simulink model "ver2_real_disc"  (R2018b)
settings: Solver=FixedStepAuto  StartTime=0.0  StopTime=10  FixedStep=10e-5  RelTol=1e-3
InitFcn:
  | ver2_real_pend_disc
values from neighbouring files (symbols this model uses):
  A_new = [A,zeros(2,1) ... (first row only)    [ver1_real_pend_cont.m]    (also in ver1_real_pendulum.m; ver2_real_pend_disc.m)
  B_new = [B ... (first row only)    [ver1_real_pend_cont.m]    (also in ver1_real_pendulum.m; ver2_real_pend_disc.m)
  E = [0 ... (first row only)    [ver1_real_pend_cont.m]    (also in ver1_real_pendulum.m; ver2_real_pend_disc.m)
  Init_condition = [0 ... (first row only)    [ver1_real_pend_cont.m]    (also in ver1_real_pendulum.m; ver2_real_pend_disc.m)
  K = lqr(A_new,B_new,Q,R)    [ver1_real_pend_cont.m]    (also in ver1_real_pendulum.m = dlqr(A_new,B_new,Q,R); ver2_real_pend_disc.m = dlqr(A_ne,B_ne,Q,R))
settings Model: Creator=Mehmet  LastModifiedBy=Seko
settings SFSimCC: SimUseLocalCustomCode=off
settings RTWCC: RTWUseLocalCustomCode=off

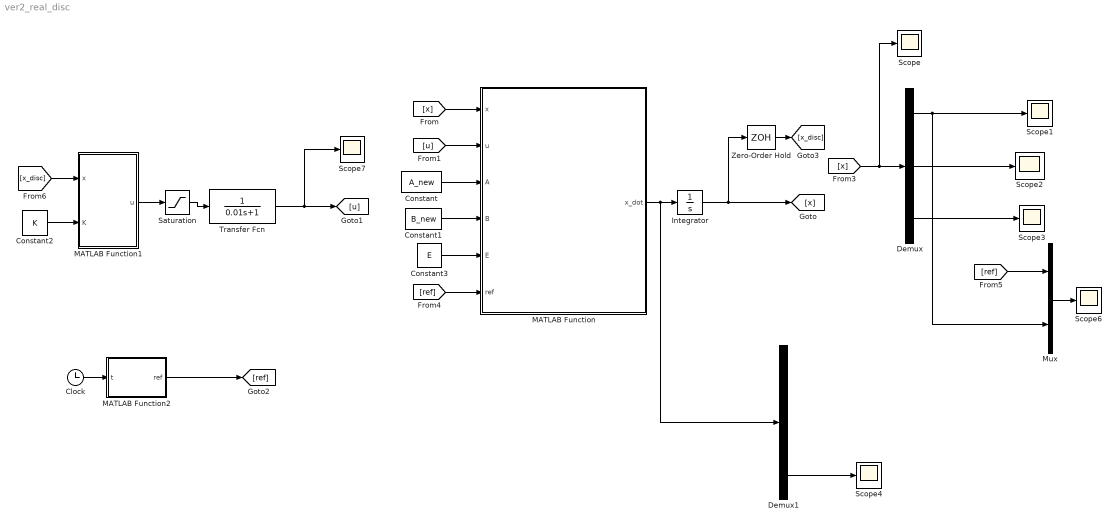
== system ver2_real_disc ==
  Clock : Clock
  Constant : Constant  Value=A_new  VectorParams1D=off
  Constant1 : Constant  Value=B_new  VectorParams1D=off
  Constant2 : Constant  Value=K  VectorParams1D=off
  Constant3 : Constant  Value=E  VectorParams1D=off
  Demux : Demux  Outputs=3
  Demux1 : Demux  Outputs=3
  Integrator : Integrator  InitialCondition=Init_condition
  MATLAB Function : MATLAB Function  TreatAsAtomicUnit=on
  MATLAB Function1 : MATLAB Function  TreatAsAtomicUnit=on
  MATLAB Function2 : MATLAB Function  TreatAsAtomicUnit=on
  Mux : Mux  Inputs=2
  Saturation : Saturate  UpperLimit=6  LowerLimit=-6
  Scope{,1..4,6..7} (7 alike) : Scope
  Transfer Fcn : TransferFcn  Denominator=[0.01 1]
  Zero-Order Hold : ZeroOrderHold  SampleTime=0.04
  wires:
  MATLAB Function/1(x_dot) -> Integrator/1, Demux1/1
  Integrator/1 -> Zero-Order Hold/1, [x]
  [x] -> MATLAB Function/1(x)
  [u] -> MATLAB Function/2(u)
  Constant/1 -> MATLAB Function/3(A)
  Constant1/1 -> MATLAB Function/4(B)
  [x_disc] -> MATLAB Function1/1(x)
  Constant2/1 -> MATLAB Function1/2(K)
  [x] -> Scope/1, Demux/1
  Demux/1 -> Mux/2, Scope1/1
  Demux/2 -> Scope2/1
  Demux/3 -> Scope3/1
  Constant3/1 -> MATLAB Function/5(E)
  Clock/1 -> MATLAB Function2/1(t)
  [ref] -> MATLAB Function/6(ref)
  [ref] -> Mux/1
  Mux/1 -> Scope6/1
  MATLAB Function1/1(u) -> Saturation/1
  MATLAB Function2/1(ref) -> [ref]
  Demux1/3 -> Scope4/1
  Saturation/1 -> Transfer Fcn/1
  Zero-Order Hold/1 -> [x_disc]
  Transfer Fcn/1 -> Scope7/1, [u]

== matlab function ver2_real_disc/MATLAB Function1 ==
  data: x input; u output; K input
function u = fcn(x,K)

u_int = -K*x;

% if abs(u_int) < (20*3.36*10^-3) && u_int > 0
% 
%     u_int = (20*3.36*10^-3);
%     
% end
% 
% if abs(u_int) < (20*3.36*10^-3) && u_int < 0
% 
%     u_int = -(20*3.36*10^-3);
%     
% end

% 
% if abs(u_int) < (20*10^-3)
% 
%     u_int = 0;
%     
% end

u = u_int;

== matlab function ver2_real_disc/MATLAB Function ==
  data: x input; u input; x_dot output; A input; B input; E input; ref input
function x_dot = fcn(x,u,A,B,E,ref)

Kt = 1.54;
torque_static = 0.20;


theta_dot = x(2,1);

x_dot_in = zeros(3,1);

% output
x_dot_in = A*x + B*u + E*ref;


if abs(Kt*u) < torque_static && theta_dot < 0.1
    
    theta_dot = 0;
    
    x_in = [x(1);theta_dot;x(3)];
    
    x_dot_in = A*x_in + B*u + E*ref;
    
end

x_dot = x_dot_in;

end

== matlab function ver2_real_disc/MATLAB Function2 ==
  data: t input; ref output
function ref = fcn(t)


f = 0.2;

A = 300*0.088*pi/180;
B = 0;

ref = A*sin(2*pi*f*t) + B;



end
